simulink model "q2section1"  (R2019a)
settings: Solver=VariableStepAuto  StartTime=0.0  StopTime=6  RelTol=1e-3
values from neighbouring files (symbols this model uses):
  A = 5*10^(-3)    (= 0.005)    [q2.m]
  beta = 10^9    (= 1000000000)    [q2.m]
  cf = 9*10^3    (= 9000)    [q2.m]
  ct = 2*10^(-10)    (= 2e-10)    [q2.m]
  dens = 850    [q2.m]
  g = 9.81    [q2.m]
  Kq = 2*10^(-3)    (= 0.002)    [q2.m]
  m = 100    [q2.m]
  mL = 1000    [q2.m]
  Ps = 7*10^6    (= 7000000)    [q2.m]
  V = 11*10^(-3)    (= 0.011)    [q2.m]
  xv_eq = (ct*m*g)/(A*Kq*sqrt((Ps-(m*g/A))/dens))    [q2.m]
settings Model: Creator=Nir Lalum  LastModifiedBy=Nir Lalum

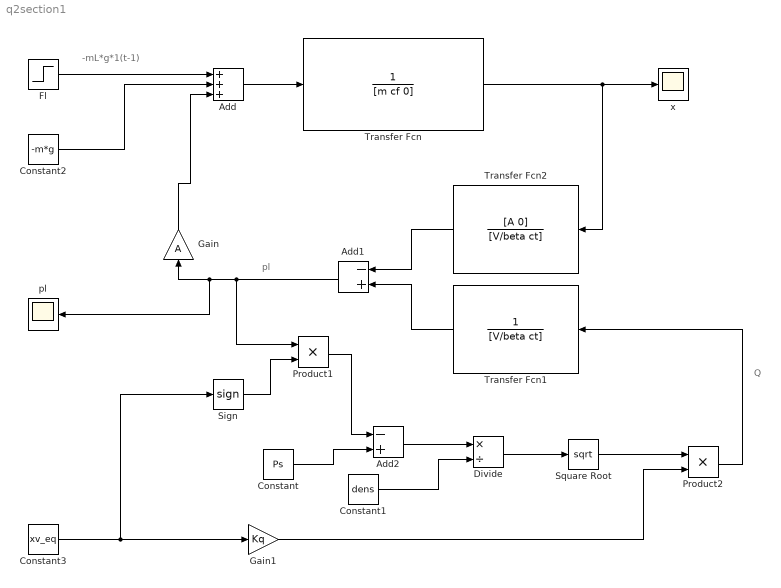
== system q2section1 ==
  note: -mL*g*1(t-1)
  note: Q
  note: pl
  Add : Sum  Inputs=+++
  Add1 : Sum  Inputs=-+
  Add2 : Sum  Inputs=-+
  Constant : Constant  Value=Ps
  Constant1 : Constant  Value=dens
  Constant2 : Constant  Value=-m*g
  Constant3 : Constant  Value=xv_eq
  Divide : Product  Inputs=*/
  Fl : Step  Before=-mL*g  After=0  SampleTime=0
  Gain : Gain  Gain=A
  Gain1 : Gain  Gain=Kq
  Product1 : Product
  Product2 : Product
  Sign : Signum
  Square Root : Sqrt  SaturateOnIntegerOverflow=on
  Transfer Fcn : TransferFcn  Denominator=[m cf 0]
  Transfer Fcn1 : TransferFcn  Denominator=[V/beta ct]
  Transfer Fcn2 : TransferFcn  Numerator=[A 0]  Denominator=[V/beta ct]
  pl : Scope
  x : Scope
  wires:
  Fl/1 -> Add/1
  Gain/1 -> Add/3
  Transfer Fcn/1 -> Transfer Fcn2/1, x/1
  Constant3/1 -> Sign/1, Gain1/1
  Constant/1 -> Add2/2
  Sign/1 -> Product1/2
  Product1/1 -> Add2/1
  Add2/1 -> Divide/1
  Constant1/1 -> Divide/2
  Divide/1 -> Square Root/1
  Square Root/1 -> Product2/1
  Gain1/1 -> Product2/2
  Product2/1 -> Transfer Fcn1/1
  Add/1 -> Transfer Fcn/1
  Add1/1 -> Product1/1, pl/1, Gain/1
  Constant2/1 -> Add/2
  Transfer Fcn2/1 -> Add1/1
  Transfer Fcn1/1 -> Add1/2
